simulink model "unidade3TestarBomba"  (R2015b)
settings: Solver=ode1  StartTime=0.0  StopTime=inf  FixedStep=0.002  RelTol=1e-3
PostLoadFcn:
  | qc_set_target_type(getConfigSet(bdroot, 'QUARC Default Target Configuration'));
undefined symbols (not defined in the file or in its folder): HIL
libraries: quarc_library x3
settings Model: SimulationMode=external  ExtModeTrigDuration=30000  Creator=MLevis  LastModifiedBy=UFRN
settings SolverCC: PositivePriorityOrder=on
settings DataIOCC: SaveFormat=Array  SignalLoggingSaveFormat=ModelDataLogs
settings OptimizationCC: ExpressionDepthLimit=2147483647  InitFltsAndDblsToZero=on
settings DebuggingCC: SaveWithParameterizedLinksMsg=none  UnderspecifiedInitializationDetection=Classic  MergeDetectMultiDrivingBlocksExec=none  SolverPrmCheckMsg=warning  MultiTaskDSMMsg=warning  MultiTaskCondExecSysMsg=none  FcnCallInpInsideContextMsg=UseLocalSettings  StateNameClashWarn=warning
settings HardwareCC: ProdBitPerPointer=32  ProdLargestAtomicFloat=None  ProdIntDivRoundTo=Undefined  ProdEndianess=Unspecified  ProdWordSize=32  ProdHWDeviceType=32-bit Generic
settings RTWCC: SystemTargetFile=quarc_win64.tlc  TemplateMakefile=quarc_default_tmf  Description=QUARC Win64 Target
settings GRTTargetCC: ParMdlRefBuildCompliant=off  CompOptLevelCompliant=off  GeneratePreprocessorConditionals=Disable all  CombineOutputUpdateFcns=off  MatFileLogging=off  GRTInterface=on  UseToolchainInfoCompliant=off  ExtMode=on  ExtModeMexFile=quarc_comm
settings ConfigComp: CovModelRefEnable=Off

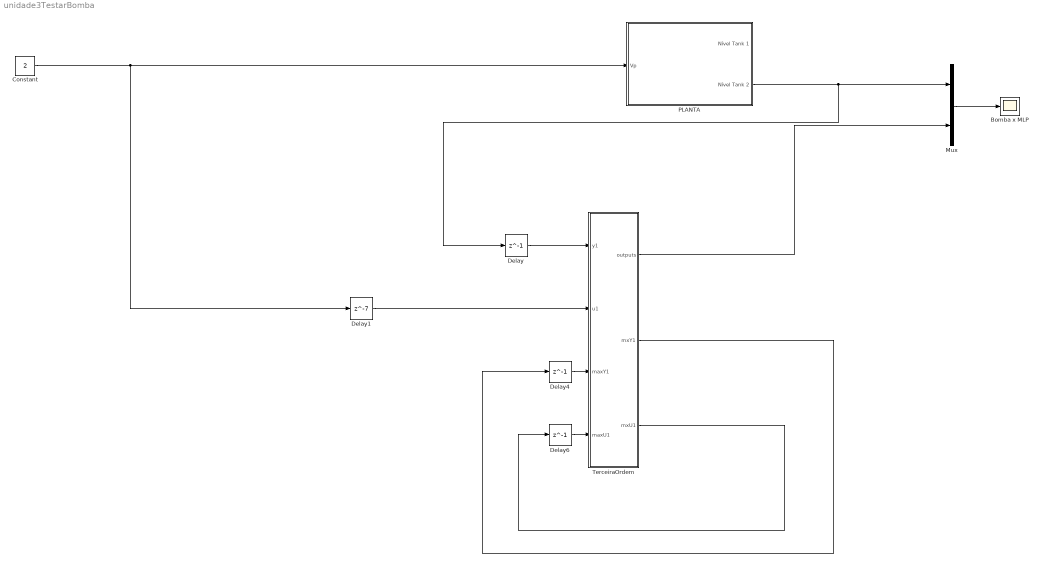
== system unidade3TestarBomba ==
  "Bomba x MLP " : Scope
  Constant : Constant  Value=2
  Delay : Delay  DelayLength=1  InitialCondition=0
  Delay1 : Delay  DelayLength=7  InitialCondition=0
  Delay4 : Delay  DelayLength=1  InitialCondition=0
  Delay6 : Delay  DelayLength=1  InitialCondition=0
  Mux : Mux  Inputs=2
  PLANTA : Subsystem
  "TerceiraOrdem " : MATLAB Function  TreatAsAtomicUnit=on
  wires:
  Mux/1 -> "Bomba x MLP "/1
  Delay/1 -> "TerceiraOrdem "/1(y1)
  Delay1/1 -> "TerceiraOrdem "/2(u1)
  PLANTA/2(Nível Tank 2) -> Delay/1, Mux/1
  Constant/1 -> Delay1/1, PLANTA/1(Vp)
  "TerceiraOrdem "/1(outputs) -> Mux/2
  "TerceiraOrdem "/2(mxY1) -> Delay4/1
  "TerceiraOrdem "/3(mxU1) -> Delay6/1
  Delay4/1 -> "TerceiraOrdem "/3(maxY1)
  Delay6/1 -> "TerceiraOrdem "/4(maxU1)

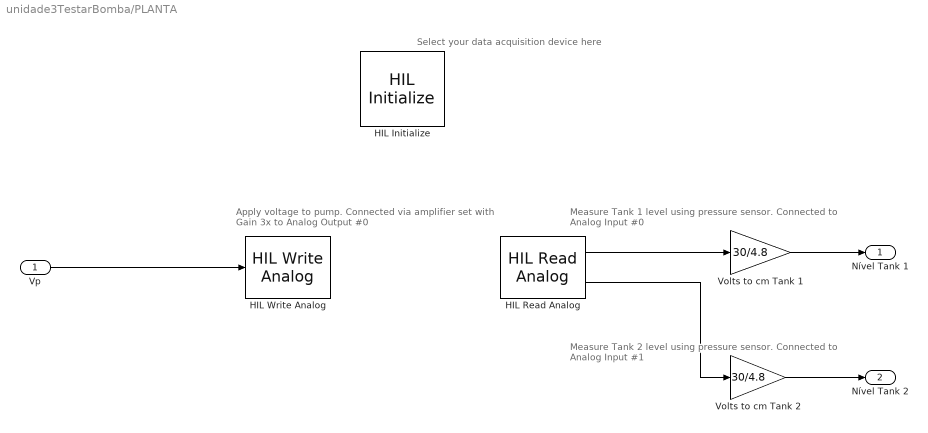
== system unidade3TestarBomba/PLANTA ==
  note: Select your data acquisition device here
  note: Apply voltage to pump.
      | Connected via amplifier set with Gain 3x
      | to  Analog Output #0
  note: Measure Tank 2 level using pressure sensor.
      | Connected to Analog Input #1
  note: Measure Tank 1 level using pressure sensor.
      | Connected to Analog Input #0
  Vp : Inport
  HIL Initialize : quarc_library/Data Acquisition/Generic/Configuration/HIL Initialize  object_name=HIL-1  board_type=q8_usb  board_number=0  board_options=update_rate=normal;decimation=1  exclusive=off  active=off  hardware_clocks=[0:2]  clock_modes=[]  initial_clock_frequencies=[]  set_clock_params_at_start=off  set_clock_params_at_switch_in=off  set_clock_frequencies_at_start=off  set_clock_frequencies_at_switch_in=off  analog_input_channels=[0:7]  analog_input_maximums=10  analog_input_minimums=-10  set_analog_input_params_at_start=on  set_analog_input_params_at_switch_in=off  analog_output_channels=[0:7]  analog_output_maximums=10  analog_output_minimums=-10  initial_analog_outputs=[0]  final_analog_outputs=[0]  watchdog_analog_outputs=0  set_analog_output_params_at_start=on  set_analog_output_params_at_switch_in=off  set_analog_outputs_at_start=on  set_analog_outputs_at_switch_in=off  set_analog_outputs_at_terminate=on  set_analog_outputs_at_switch_out=off  set_analog_outputs_on_watchdog=off  digital_input_channels=[]  digital_output_channels=[]  digital_output_configuration=[]  initial_digital_outputs=[1]  final_digital_outputs=[1]  watchdog_digital_outputs=[1]  set_digital_output_params_at_start=off  set_digital_output_params_at_switch_in=off  set_digital_outputs_at_start=on  set_digital_outputs_at_switch_in=off  set_digital_outputs_at_terminate=on  set_digital_outputs_at_switch_out=off  set_digital_outputs_on_watchdog=off  encoder_channels=[0:7]  quadrature=[4]  encoder_filter_frequency=[]  initial_encoder_counts=[0]  set_encoder_params_at_start=on  set_encoder_params_at_switch_in=off  set_encoder_counts_at_start=on  set_encoder_counts_at_switch_in=off  pwm_channels=[0:7]  pwm_modes=0  pwm_frequency=99.532799999999995e6/4095  pwm_configuration=[0]  pwm_alignment=[0]  pwm_polarity=[1]  pwm_leading_deadband=[0]  pwm_trailing_deadband=[0]  initial_pwm_outputs=[0]  final_pwm_outputs=[0]  watchdog_pwm_outputs=[0]  set_pwm_params_at_start=on  set_pwm_params_at_switch_in=off  set_pwm_outputs_at_start=on  set_pwm_outputs_at_switch_in=off  set_pwm_outputs_at_terminate=on  set_pwm_outputs_at_switch_out=off  set_pwm_outputs_on_watchdog=off  other_output_channels=[]  initial_other_outputs=[]  final_other_outputs=[]  watchdog_other_outputs=[]  set_other_outputs_at_start=off  set_other_outputs_at_switch_in=off  set_other_outputs_at_terminate=off  set_other_outputs_at_switch_out=off  set_other_outputs_on_watchdog=off
  HIL Read Analog : quarc_library/Data Acquisition/Generic/Immediate I//O/HIL Read Analog  object_name=HIL-1  channels=[0:1]  sample_time=qc_get_step_size  active=on  vector_output=off
  HIL Write Analog : quarc_library/Data Acquisition/Generic/Immediate I//O/HIL Write Analog  object_name=HIL-1  channels=0  sample_time=-1  active=off  vector_input=off
  "Volts to cm Tank 1 " : Gain  Gain=30/4.8
  Volts to cm Tank 2 : Gain  Gain=30/4.8
  Nível Tank 1 : Outport
  Nível Tank 2 : Outport  Port=2
  wires:
  HIL Read Analog/1 -> "Volts to cm Tank 1 "/1
  HIL Read Analog/2 -> Volts to cm Tank 2/1
  Vp/1 -> HIL Write Analog/1
  "Volts to cm Tank 1 "/1 -> Nível Tank 1/1
  Volts to cm Tank 2/1 -> Nível Tank 2/1

== matlab function unidade3TestarBomba/TerceiraOrdem  ==
  data: y1 input; u1 input; outputs output; maxY1 input; maxU1 input; mxY1 output; mxU1 output
%% Ordem 1, Atraso 1
function [outputs,mxY1,mxU1] = EvaluateNetworkForSimulink(y1,u1,maxY1,maxU1)
%nbrOfLayers = length(nce);
PesosIn=[ -0.0328    0.4559   -0.7624    0.8638    0.5223    0.3606    0.8657   -0.4199   -0.4578   -0.0453    0.7853   -0.7235    0.7825    0.4438   -0.0620   -0.1569    0.5046   -0.1227   -0.6142	-0.5768 0.9509;
    0.0497    1.0016    0.2246   -0.1089    0.0416   -1.0625   -0.3390    0.0020    0.8252   -0.5963   -0.7131    0.6855   -1.0542   -0.8804    0.8025    0.0814   -0.4549    0.0089   -0.7778   -1.1001	1.1030;
    0.0100   -0.5080   -0.1506   -0.2785   -0.8003   -0.4934   -0.0855    0.2045   -0.9185   -0.0646    0.3636   -0.8672   -1.0282    0.4316   -0.4392    0.2075   -0.0972    1.0112    0.9569    0.6910    0.4716];


PesosEsc=[0.1576;
    0.5431;
    0.1525;
    0.0141;
   -0.0364;
   -0.60140;
   -0.0766;
    0.1122;
    0.3645;
   -0.2741;
   -0.2142;
    0.2881;
   -0.6810;
   -0.3277;
    0.4723;
    0.1724;
   -0.1802;
    0.2843;
   -0.1379;
   -0.3472;
    0.5732];


PesosOut=1;



maxY1=max(maxY1,y1);
maxU1=max(maxU1,u1);


y1=y1./maxY1;
u1=u1./maxU1;


Sample=[y1 u1];
Sample = [ones(length(Sample(:,1)),1) Sample];

NodeIn = Sample;

NodeIn = NodeIn*PesosIn;



NodeIn = FuncaoAtivacao(NodeIn,'LOGSIGMOIDE');

NodeHid=NodeIn;


NodeHid = NodeHid*PesosEsc;

NodeHid = FuncaoAtivacao(NodeHid,'LOGSIGMOIDE');


NodeOut=NodeHid;
NodeOut = NodeOut*PesosOut;

outputs=NodeOut.*max(maxY1,maxU1);

mxY1=maxY1;
mxU1=maxU1;

end
